simulink model "RocketSimForArchitecture"  (R2024b)
settings: Solver=VariableStepAuto  StartTime=0.0  StopTime=10.0  RelTol=1e-3  AbsTol=1e-3
model workspace (MAT data in the model file):
  m = 1
values from neighbouring files (symbols this model uses):
  X =     [ga_pid_best_result.mat]    (also in pid_vals.mat)
  Y =     [ga_pid_best_result.mat]    (also in pid_vals.mat)
  Z =     [ga_pid_best_result.mat]    (also in pid_vals.mat)
libraries: fl_lib x25, nesl_utility x22, sm_lib x12, ee_lib x9, slpidlib x4, matrix_library x2, aerolibutil x2, sdl_lib x1, shared6dof x1, robotcorelib x1, aerolibnav x1
(part 2 of 2)

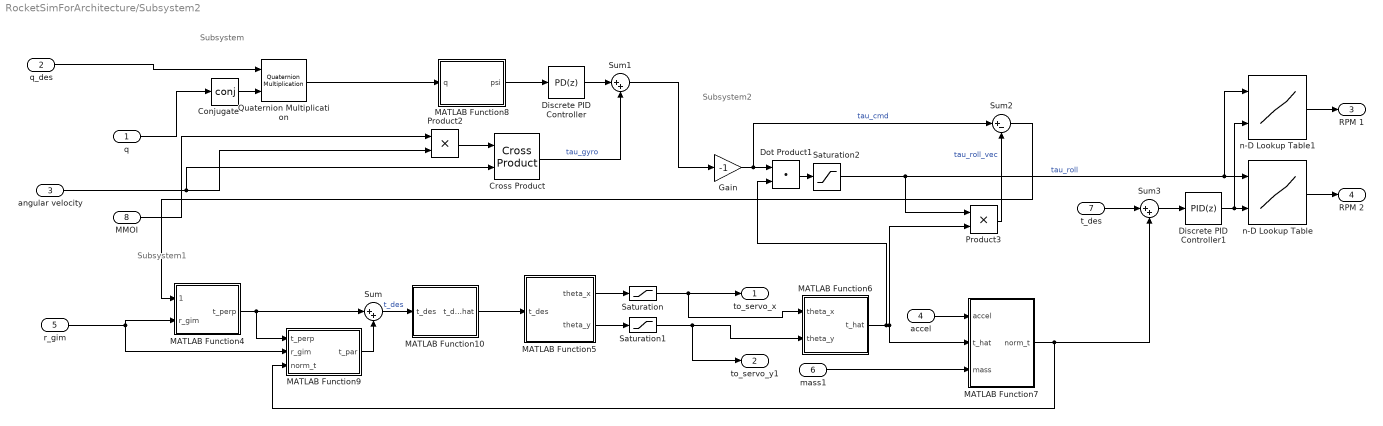
== system RocketSimForArchitecture/Subsystem2 ==
  note: Subsystem1
  note: Subsystem
  note: Subsystem2
  q : Inport  PortDimensions=4
  q_des : Inport  Port=2  PortDimensions=4
  angular velocity : Inport  Port=3  PortDimensions=3
  accel : Inport  Port=4  PortDimensions=3
  r_gim : Inport  Port=5  PortDimensions=3
  mass1 : Inport  Port=6  PortDimensions=1
  t_des : Inport  Port=7  PortDimensions=3
  MMOI : Inport  Port=8
  Conjugate : Math  Operator=conj  SignedPower=on  RndMeth=Zero
  Cross Product : matrix_library/Cross Product
  Discrete PID Controller : slpidlib/PID Controller  Controller=PD  Form=Parallel  TimeDomain=Discrete-time  UseExternalTs=off  SampleTime=0.001  IntegratorMethod=Forward Euler  FilterMethod=Forward Euler  ControllerParametersSource=internal  P=1  I=1  UseKiTs=off  D=1  UseExternalDerivativeSource=off  N=1  UseFilter=on  TunerSelectOption=Transfer Function Based (PID Tuner App)  InitialConditionSource=internal  InitialConditionForIntegrator=0  InitialConditionForFilter=1  DifferentiatorICPrevScaledInput=0  ExternalReset=none  TrackingMode=off  Kt=1  LimitOutput=on  SatLimitsSource=internal  UpperSaturationLimit=10  LowerSaturationLimit=-10  LinearizeAsGain=off  AntiWindupMode=none  Kb=1  LimitIntegrator=off  UpperIntegratorSaturationLimit=inf  LowerIntegratorSaturationLimit=-inf  POutMin=[]  POutMax=[]  IOutMin=[]  IOutMax=[]  DOutMin=[]  DOutMax=[]  NOutMin=[]  NOutMax=[]  SumOutMin=[]  SumOutMax=[]  SaturationOutMin=[]  SaturationOutMax=[]  PParamMin=[]  PParamMax=[]  IParamMin=[]  IParamMax=[]  DParamMin=[]  DParamMax=[]  NParamMin=[]  NParamMax=[]  KbParamMin=[]  KbParamMax=[]  KtParamMin=[]  KtParamMax=[]  KbOutMin=[]  KbOutMax=[]  KtOutMin=[]  KtOutMax=[]  IntegratorOutMin=[]  IntegratorOutMax=[]  FilterOutMin=[]  FilterOutMax=[]  SumI1OutMin=[]  SumI1OutMax=[]  SumI2OutMin=[]  SumI2OutMax=[]  SumI3OutMin=[]  SumI3OutMax=[]  SumI4OutMin=[]  SumI4OutMax=[]  SumDOutMin=[]  SumDOutMax=[]  DifferentiatorOutMin=[]  DifferentiatorOutMax=[]  FilterDiffOutCoefMin=[]  FilterDiffOutCoefMax=[]  ReciprocalOutMin=[]  ReciprocalOutMax=[]  SumDenOutMin=[]  SumDenOutMax=[]  SumNumOutMin=[]  SumNumOutMax=[]  DivideOutMin=[]  DivideOutMax=[]  UdiffTsProdOutMin=[]  UdiffTsProdOutMax=[]  NTsProdOutMin=[]  NTsProdOutMax=[]  UintegralTsProdOutMin=[]  UintegralTsProdOutMax=[]  UngainTsProdOutMin=[]  UngainTsProdOutMax=[]  ClampingZeroOutDataTypeStr=Inherit: Inherit via back propagation  ClampingZeroOutMin=[]  ClampingZeroOutMax=[]  FilterDenConstantOutDataTypeStr=Inherit: Inherit via back propagation  FilterDenConstantOutMin=[]  FilterDenConstantOutMax=[]  PCopyOutDataTypeStr=Inherit: Inherit via back propagation  PCopyOutMin=[]  PCopyOutMax=[]  NCopyOutDataTypeStr=Inherit: Inherit via back propagation  NCopyOutMin=[]  NCopyOutMax=[]  IntegratorContinuousStateAttributes=''  IntegratorStateMustResolveToSignalObject=off  IntegratorRTWStateStorageClass=Auto  FilterContinuousStateAttributes=''  FilterStateMustResolveToSignalObject=off  FilterRTWStateStorageClass=Auto  ParallelPVariant=InternalParameters  IdealPVariant=Disabled  IVariant=Disabled  DVariant=InternalParameters  IntegratorVariant=Disabled  SatVariant=Enabled  AWVariant=Disabled  PCopyVariant=Disabled  TRVariant=Disabled  FdbkBlocksVariant=Forward  IdealPFdbkVariant=Disabled  SatFdbkVariant=Disabled  DerivativeFilterVariant=ForwardEulerFilter  NVariant=InternalParameters  NCopyVariant=Disabled  FilterICVariant=InternalICsFilter  IntegratorICVariant=Disabled  ExternalResetVariant=Disabled  TRSumVariant=Passthrough  SumFdbkVariant=Disabled  SumVariant=Sum_PD  TsampFilterVariant=InternalTs  TsampNgainVariant=Passthrough  TsampIntegralVariant=Disabled_SignalSpec  ExternalSaturationOutDataTypeStr=Inherit: Same as second input  DerivativeSourceVariant=ErrorSignal  PreIntVariant=InternalPreInt
  Discrete PID Controller1 : slpidlib/PID Controller  Controller=PID  Form=Parallel  TimeDomain=Discrete-time  UseExternalTs=off  SampleTime=0.001  IntegratorMethod=Forward Euler  FilterMethod=Forward Euler  ControllerParametersSource=internal  P=0  I=1  UseKiTs=off  D=1  UseExternalDerivativeSource=off  N=100  UseFilter=on  TunerSelectOption=Transfer Function Based (PID Tuner App)  InitialConditionSource=internal  InitialConditionForIntegrator=0  InitialConditionForFilter=0  DifferentiatorICPrevScaledInput=0  ExternalReset=none  TrackingMode=off  Kt=1  LimitOutput=off  SatLimitsSource=internal  UpperSaturationLimit=inf  LowerSaturationLimit=-inf  LinearizeAsGain=off  AntiWindupMode=none  Kb=1  LimitIntegrator=off  UpperIntegratorSaturationLimit=inf  LowerIntegratorSaturationLimit=-inf  POutMin=[]  POutMax=[]  IOutMin=[]  IOutMax=[]  DOutMin=[]  DOutMax=[]  NOutMin=[]  NOutMax=[]  SumOutMin=[]  SumOutMax=[]  SaturationOutMin=[]  SaturationOutMax=[]  PParamMin=[]  PParamMax=[]  IParamMin=[]  IParamMax=[]  DParamMin=[]  DParamMax=[]  NParamMin=[]  NParamMax=[]  KbParamMin=[]  KbParamMax=[]  KtParamMin=[]  KtParamMax=[]  KbOutMin=[]  KbOutMax=[]  KtOutMin=[]  KtOutMax=[]  IntegratorOutMin=[]  IntegratorOutMax=[]  FilterOutMin=[]  FilterOutMax=[]  SumI1OutMin=[]  SumI1OutMax=[]  SumI2OutMin=[]  SumI2OutMax=[]  SumI3OutMin=[]  SumI3OutMax=[]  SumI4OutMin=[]  SumI4OutMax=[]  SumDOutMin=[]  SumDOutMax=[]  DifferentiatorOutMin=[]  DifferentiatorOutMax=[]  FilterDiffOutCoefMin=[]  FilterDiffOutCoefMax=[]  ReciprocalOutMin=[]  ReciprocalOutMax=[]  SumDenOutMin=[]  SumDenOutMax=[]  SumNumOutMin=[]  SumNumOutMax=[]  DivideOutMin=[]  DivideOutMax=[]  UdiffTsProdOutMin=[]  UdiffTsProdOutMax=[]  NTsProdOutMin=[]  NTsProdOutMax=[]  UintegralTsProdOutMin=[]  UintegralTsProdOutMax=[]  UngainTsProdOutMin=[]  UngainTsProdOutMax=[]  ClampingZeroOutDataTypeStr=Inherit: Inherit via back propagation  ClampingZeroOutMin=[]  ClampingZeroOutMax=[]  FilterDenConstantOutDataTypeStr=Inherit: Inherit via back propagation  FilterDenConstantOutMin=[]  FilterDenConstantOutMax=[]  PCopyOutDataTypeStr=Inherit: Inherit via back propagation  PCopyOutMin=[]  PCopyOutMax=[]  NCopyOutDataTypeStr=Inherit: Inherit via back propagation  NCopyOutMin=[]  NCopyOutMax=[]  IntegratorContinuousStateAttributes=''  IntegratorStateMustResolveToSignalObject=off  IntegratorRTWStateStorageClass=Auto  FilterContinuousStateAttributes=''  FilterStateMustResolveToSignalObject=off  FilterRTWStateStorageClass=Auto  ParallelPVariant=InternalParameters  IdealPVariant=Disabled  IVariant=InternalParameters  DVariant=InternalParameters  IntegratorVariant=Discrete  SatVariant=Disabled  AWVariant=Passthrough  PCopyVariant=Disabled  TRVariant=Disabled  FdbkBlocksVariant=Forward  IdealPFdbkVariant=Disabled  SatFdbkVariant=Disabled  DerivativeFilterVariant=ForwardEulerFilter  NVariant=InternalParameters  NCopyVariant=Disabled  FilterICVariant=InternalICsFilter  IntegratorICVariant=InternalICs  ExternalResetVariant=Disabled  TRSumVariant=Passthrough  SumFdbkVariant=Disabled  SumVariant=Sum_PID  TsampFilterVariant=InternalTs  TsampNgainVariant=Passthrough  TsampIntegralVariant=Disabled_SignalSpec  ExternalSaturationOutDataTypeStr=Inherit: Same as second input  DerivativeSourceVariant=ErrorSignal  PreIntVariant=InternalPreInt
  Dot Product1 : DotProduct  OutDataTypeStr=Inherit: Inherit via internal rule
  Gain : Gain  Gain=-1
  MATLAB Function10 : MATLAB Function  TreatAsAtomicUnit=on
  MATLAB Function4 : MATLAB Function  TreatAsAtomicUnit=on
  MATLAB Function5 : MATLAB Function  TreatAsAtomicUnit=on
  MATLAB Function6 : MATLAB Function  TreatAsAtomicUnit=on
  MATLAB Function7 : MATLAB Function  TreatAsAtomicUnit=on
  MATLAB Function8 : MATLAB Function  TreatAsAtomicUnit=on
  MATLAB Function9 : MATLAB Function  TreatAsAtomicUnit=on
  Product2 : Product
  Product3 : Product
  Quaternion Multiplication : aerolibutil/Quaternion Multiplication
  Saturation : Saturate
  Saturation1 : Saturate
  Saturation2 : Saturate
  Sum : Sum  Inputs=|++
  Sum1 : Sum  Inputs=|++
  Sum2 : Sum  Inputs=|+-
  Sum3 : Sum  Inputs=|++
  n-D Lookup Table : Lookup_n-D  LookupTableObject=''  BreakpointsForDimension1=[1:2]  BreakpointsForDimension2=[1:2]  BreakpointsForDimension3=[5, 7]  BreakpointsForDimension1FirstPoint=10  BreakpointsForDimension2FirstPoint=10  BreakpointsForDimension1Spacing=12  BreakpointsForDimension2Spacing=12  IndexSearchMethod=Evenly spaced points  Table=[4 5;16 19]  InterpMethod=Flat  DiagnosticForOutOfRangeInput=Error  InternalRulePriority=Speed  RndMeth=Simplest
      settings: InputPortMap=u0,u1
  n-D Lookup Table1 : Lookup_n-D  LookupTableObject=''  BreakpointsForDimension1=[1:2]  BreakpointsForDimension2=[1:2]  BreakpointsForDimension3=[5, 7]  BreakpointsForDimension1FirstPoint=10  BreakpointsForDimension2FirstPoint=10  BreakpointsForDimension1Spacing=12  BreakpointsForDimension2Spacing=12  IndexSearchMethod=Evenly spaced points  Table=[4 5;16 19]  InterpMethod=Flat  DiagnosticForOutOfRangeInput=Error  InternalRulePriority=Speed  RndMeth=Simplest
      settings: InputPortMap=u0,u1
  to_servo_x : Outport  PortDimensions=1
  to_servo_y1 : Outport  Port=2  PortDimensions=1
  RPM 1 : Outport  Port=3
  RPM 2 : Outport  Port=4
  wires:
  Discrete PID Controller1/1 -> n-D Lookup Table1/2, n-D Lookup Table/2
  Conjugate/1 -> Quaternion Multiplication/2
  MATLAB Function5/1(theta_x) -> Saturation/1
  Quaternion Multiplication/1 -> MATLAB Function8/1(q)
  Gain/1 -> Sum2/1, Dot Product1/1  "tau_cmd"
  n-D Lookup Table/1 -> RPM 2/1
  Saturation1/1 -> to_servo_y1/1, MATLAB Function6/2(theta_y)
  Sum/1 -> MATLAB Function10/1(t_des)  "t_des"
  Saturation/1 -> to_servo_x/1, MATLAB Function6/1(theta_x)
  Dot Product1/1 -> Saturation2/1
  accel/1 -> MATLAB Function7/1(accel)
  Cross Product/1 -> Sum1/2  "tau_gyro"
  MATLAB Function6/1(t_hat) -> Product3/2, MATLAB Function7/2(t_hat), Dot Product1/2
  MMOI/1 -> Product2/1
  Sum2/1 -> MATLAB Function4/1(tau_gim)
  MATLAB Function4/1(t_perp) -> MATLAB Function9/1(t_perp), Sum/1
  mass1/1 -> MATLAB Function7/3(mass)
  MATLAB Function10/1(t_des_hat) -> MATLAB Function5/1(t_des)
  MATLAB Function5/2(theta_y) -> Saturation1/1
  r_gim/1 -> MATLAB Function9/2(r_gim), MATLAB Function4/2(r_gim)
  q_des/1 -> Quaternion Multiplication/1
  Saturation2/1 -> n-D Lookup Table1/1, n-D Lookup Table/1, Product3/1  "tau_roll"
  angular velocity/1 -> Product2/2, Cross Product/2
  MATLAB Function8/1(psi) -> Discrete PID Controller/1
  MATLAB Function7/1(norm_t) -> MATLAB Function9/3(norm_t), Sum3/2
  Product3/1 -> Sum2/2  "tau_roll_vec"
  Sum1/1 -> Gain/1
  Sum3/1 -> Discrete PID Controller1/1
  q/1 -> Conjugate/1
  Discrete PID Controller/1 -> Sum1/1
  MATLAB Function9/1(t_par) -> Sum/2
  Product2/1 -> Cross Product/1
  t_des/1 -> Sum3/1
  n-D Lookup Table1/1 -> RPM 1/1

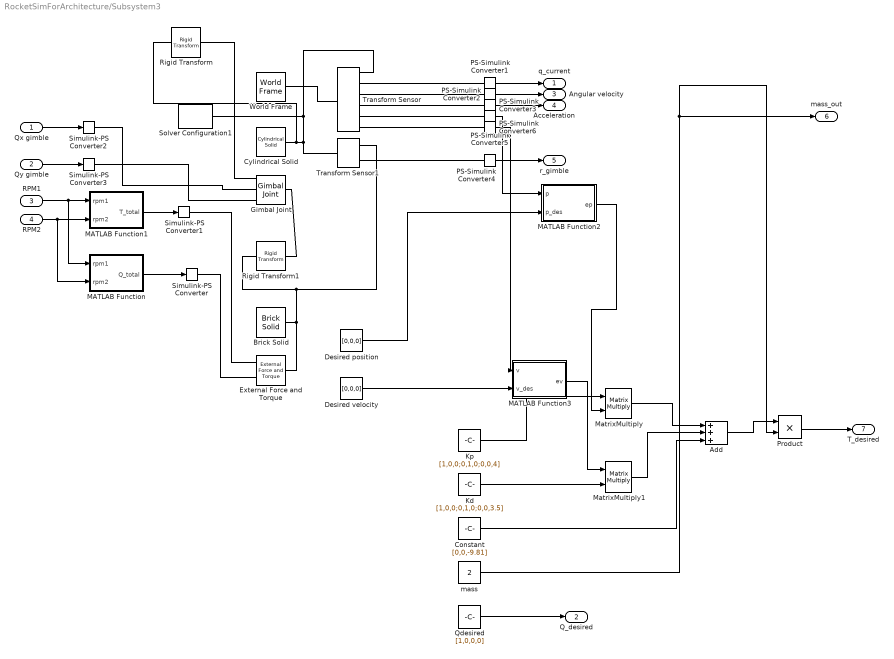
== system RocketSimForArchitecture/Subsystem3 ==
  Qx gimble : Inport
  Qy gimble : Inport  Port=2
  RPM1 : Inport  Port=3
  RPM2 : Inport  Port=4
  Add : Sum  Inputs=+++
  Brick Solid : sm_lib/Body Elements/Brick Solid  BrickDimensions=[0.1 0.1 0.2]  BrickDimensionsUnits=m  ExportEntireGeometry=off  InertiaType=CalculateFromGeometry  BasedOnType=Mass  Density=1000  DensityUnits=kg/m^3  Mass=0.5  MassUnits=kg  CenterOfMass=[0 0 0]  CenterOfMassUnits=m  MomentsOfInertia=[1 1 1]  MomentsOfInertiaUnits=kg*m^2  ProductsOfInertia=[0 0 0]  ProductsOfInertiaUnits=kg*m^2  GraphicType=FromGeometry  MarkerShape=Sphere  MarkerSize=10  GraphicVisPropType=SimpleVisualProperties  GraphicDiffuseColor=[1 0 0]  GraphicOpacity=1  GraphicSpecularColor=[0.5 0.5 0.5 1.0]  GraphicAmbientColor=[0.15 0.15 0.15 1.0]  GraphicEmissiveColor=[0.0 0.0 0.0 1.0]  GraphicShininess=75  DoExposeReferenceFrame=on  SerializedFrames=<Frames/>
  Constant : Constant  Value=[0,0,-9.81]
  Cylindrical Solid : sm_lib/Body Elements/Cylindrical Solid  CylinderRadius=0.08  CylinderRadiusUnits=m  CylinderLength=0.4  CylinderLengthUnits=m  ExportEntireGeometry=off  InertiaType=CalculateFromGeometry  BasedOnType=Mass  Density=1.5  DensityUnits=kg/m^3  Mass=1.5  MassUnits=kg  CenterOfMass=[0 0 0]  CenterOfMassUnits=m  MomentsOfInertia=[1 1 1]  MomentsOfInertiaUnits=kg*m^2  ProductsOfInertia=[0 0 0]  ProductsOfInertiaUnits=kg*m^2  GraphicType=FromGeometry  MarkerShape=Sphere  MarkerSize=10  GraphicVisPropType=SimpleVisualProperties  GraphicDiffuseColor=[0 0.4471 0.7412]  GraphicOpacity=1  GraphicSpecularColor=[0.5 0.5 0.5 1.0]  GraphicAmbientColor=[0.15 0.15 0.15 1.0]  GraphicEmissiveColor=[0.0 0.0 0.0 1.0]  GraphicShininess=75  DoExposeReferenceFrame=on  SerializedFrames=<Frames/>
  Desired position : Constant  Value=[0,0,0]
  Desired velocity : Constant  Value=[0,0,0]
  External Force and Torque : sm_lib/Forces and Torques/External Force and Torque  EnableForceX=off  EnableForceY=off  EnableForceZ=on  EnableForce=off  ForceResolutionFrame=AttachedFrame  EnableTorqueX=off  EnableTorqueY=off  EnableTorqueZ=on  EnableTorque=off  TorqueResolutionFrame=AttachedFrame
  Gimbal Joint : sm_lib/Joints/Gimbal Joint  JointMode=Normal  CompositeWrenchDir=FollowerOnBase  CompositeWrenchFrame=BaseFrame  SenseConstraintForce=off  SenseConstraintTorque=off  SenseTotalForce=off  SenseTotalTorque=off  RxPositionTargetSpecify=off  RxPositionTargetPriority=High  RxPositionTargetValue=0  RxPositionTargetValueUnits=deg  RxVelocityTargetSpecify=off  RxVelocityTargetPriority=High  RxVelocityTargetValue=0  RxVelocityTargetValueUnits=deg/s  RxEquilibriumPosition=0  RxEquilibriumPositionUnits=deg  RxSpringStiffness=0  RxSpringStiffnessUnits=N*m/deg  RxDampingCoefficient=0  RxDampingCoefficientUnits=N*m/(deg/s)  RxLowerLimitSpecify=off  RxLowerLimitBound=-90  RxLowerLimitBoundUnits=deg  RxLowerLimitStiffness=1e4  RxLowerLimitStiffnessUnits=N*m/deg  RxLowerLimitDamping=10  RxLowerLimitDampingUnits=N*m/(deg/s)  RxLowerLimitTransitionRegionWidth=0.1  RxLowerLimitTransitionRegionWidthUnits=deg  RxUpperLimitSpecify=off  RxUpperLimitBound=90  RxUpperLimitBoundUnits=deg  RxUpperLimitStiffness=1e4  RxUpperLimitStiffnessUnits=N*m/deg  RxUpperLimitDamping=10  RxUpperLimitDampingUnits=N*m/(deg/s)  RxUpperLimitTransitionRegionWidth=0.1  RxUpperLimitTransitionRegionWidthUnits=deg  RxTorqueActuationMode=ComputedTorque  RxMotionActuationMode=InputMotion  RxSensePosition=off  RxSenseVelocity=off  RxSenseAcceleration=off  RxSenseTorqueForce=off  RxSenseLowerLimitTorqueForce=off  RxSenseUpperLimitTorqueForce=off  RyPositionTargetSpecify=off  RyPositionTargetPriority=High  RyPositionTargetValue=0  RyPositionTargetValueUnits=deg  RyVelocityTargetSpecify=off  RyVelocityTargetPriority=High  RyVelocityTargetValue=0  RyVelocityTargetValueUnits=deg/s  RyEquilibriumPosition=0  RyEquilibriumPositionUnits=deg  RySpringStiffness=0  RySpringStiffnessUnits=N*m/deg  RyDampingCoefficient=0  RyDampingCoefficientUnits=N*m/(deg/s)  RyLowerLimitSpecify=off  RyLowerLimitBound=-90  RyLowerLimitBoundUnits=deg  RyLowerLimitStiffness=1e4  RyLowerLimitStiffnessUnits=N*m/deg  RyLowerLimitDamping=10  RyLowerLimitDampingUnits=N*m/(deg/s)  RyLowerLimitTransitionRegionWidth=0.1  RyLowerLimitTransitionRegionWidthUnits=deg  RyUpperLimitSpecify=off  RyUpperLimitBound=90  RyUpperLimitBoundUnits=deg  RyUpperLimitStiffness=1e4  RyUpperLimitStiffnessUnits=N*m/deg  RyUpperLimitDamping=10  RyUpperLimitDampingUnits=N*m/(deg/s)  RyUpperLimitTransitionRegionWidth=0.1  RyUpperLimitTransitionRegionWidthUnits=deg  RyTorqueActuationMode=NoTorque  RyMotionActuationMode=InputMotion  RySensePosition=off  RySenseVelocity=off  RySenseAcceleration=off  RySenseTorqueForce=off  RySenseLowerLimitTorqueForce=off  RySenseUpperLimitTorqueForce=off  RzPositionTargetSpecify=off  RzPositionTargetPriority=High  RzPositionTargetValue=0  RzPositionTargetValueUnits=deg  RzVelocityTargetSpecify=off  RzVelocityTargetPriority=High  RzVelocityTargetValue=0  RzVelocityTargetValueUnits=deg/s  RzEquilibriumPosition=0  RzEquilibriumPositionUnits=deg  RzSpringStiffness=0  RzSpringStiffnessUnits=N*m/deg  RzDampingCoefficient=0  RzDampingCoefficientUnits=N*m/(deg/s)  RzLowerLimitSpecify=off  RzLowerLimitBound=-90  RzLowerLimitBoundUnits=deg  RzLowerLimitStiffness=1e4  RzLowerLimitStiffnessUnits=N*m/deg  RzLowerLimitDamping=10  RzLowerLimitDampingUnits=N*m/(deg/s)  RzLowerLimitTransitionRegionWidth=0.1  RzLowerLimitTransitionRegionWidthUnits=deg  RzUpperLimitSpecify=off  RzUpperLimitBound=90  RzUpperLimitBoundUnits=deg  RzUpperLimitStiffness=1e4  RzUpperLimitStiffnessUnits=N*m/deg  RzUpperLimitDamping=10  RzUpperLimitDampingUnits=N*m/(deg/s)  RzUpperLimitTransitionRegionWidth=0.1  RzUpperLimitTransitionRegionWidthUnits=deg  RzTorqueActuationMode=NoTorque  RzMotionActuationMode=ComputedMotion  RzSensePosition=off  RzSenseVelocity=off  RzSenseAcceleration=off  RzSenseTorqueForce=off  RzSenseLowerLimitTorqueForce=off  RzSenseUpperLimitTorqueForce=off
  Kd : Constant  Value=[1,0,0;0,1,0;0,0,3.5]
  Kp : Constant  Value=[1,0,0;0,1,0;0,0,4]
  MATLAB Function : MATLAB Function  TreatAsAtomicUnit=on
  MATLAB Function1 : MATLAB Function  TreatAsAtomicUnit=on
  MATLAB Function2 : MATLAB Function  TreatAsAtomicUnit=on
  MATLAB Function3 : MATLAB Function  TreatAsAtomicUnit=on
  MatrixMultiply : Product  Multiplication=Matrix(*)
  MatrixMultiply1 : Product  Multiplication=Matrix(*)
  PS-Simulink Converter{1..6} (6 alike) : nesl_utility/PS-Simulink Converter  PhysicalDomain=network_engine_domain  SubClassName=ps_output  LeftPortType=input  RightPortType=output  PseudoPeriodic=off  Frequencies=[]  VectorFormat=inherit  Unit=inherit  AffineConversion=off
  Product : Product
  Qdesired : Constant  Value=[1,0,0,0]
  Rigid Transform : sm_lib/Frames and Transforms/Rigid Transform  RotationMethod=None  FollAlignAxisA=+X  BaseAlignAxisA=+Y  FollAlignAxisB=+Y  BaseAlignAxisB=+Z  RotationStandardAxis=+Z  RotationAngle=0  RotationAngleUnits=deg  RotationArbitraryAxis=[0 0 1]  RotationSequenceAxes=FollowerAxes  RotationSequence=XYX  RotationSequenceAngles=[0 0 0]  RotationSequenceAnglesUnits=deg  RotationMatrix=[1 0 0;0 1 0;0 0 1]  Quaternion=[1 0 0 0]  TranslationMethod=Cartesian  TranslationCartesianOffset=[0 0 -0.2]  TranslationCartesianOffsetUnits=m  TranslationStandardAxis=+Z  TranslationStandardOffset=0  TranslationStandardOffsetUnits=m  TranslationROffset=0  TranslationROffsetUnits=m  TranslationThetaOffset=0  TranslationThetaOffsetUnits=deg  TranslationZOffset=0  TranslationZOffsetUnits=m
  Rigid Transform1 : sm_lib/Frames and Transforms/Rigid Transform  RotationMethod=None  FollAlignAxisA=+X  BaseAlignAxisA=+Y  FollAlignAxisB=+Y  BaseAlignAxisB=+Z  RotationStandardAxis=+Z  RotationAngle=0  RotationAngleUnits=deg  RotationArbitraryAxis=[0 0 1]  RotationSequenceAxes=FollowerAxes  RotationSequence=XYX  RotationSequenceAngles=[0 0 0]  RotationSequenceAnglesUnits=deg  RotationMatrix=[1 0 0;0 1 0;0 0 1]  Quaternion=[1 0 0 0]  TranslationMethod=Cartesian  TranslationCartesianOffset=[0 0 0.1]  TranslationCartesianOffsetUnits=m  TranslationStandardAxis=+Z  TranslationStandardOffset=0  TranslationStandardOffsetUnits=m  TranslationROffset=0  TranslationROffsetUnits=m  TranslationThetaOffset=0  TranslationThetaOffsetUnits=deg  TranslationZOffset=0  TranslationZOffsetUnits=m
  Simulink-PS Converter{,1..3} (4 alike) : nesl_utility/Simulink-PS Converter  PhysicalDomain=network_engine_domain  SubClassName=ps_input  LeftPortType=input  RightPortType=output  PseudoPeriodic=off  Frequencies=[]  NoiseDistribution=none  NoiseParameters=[]  Unit=1  AffineConversion=off  FilteringAndDerivatives=provide  SimscapeFilterOrder=1  InputFilterTimeConstant=0.001  UdotUserProvided=0
  Solver Configuration1 : nesl_utility/Solver Configuration  PhysicalDomain=network_engine_domain  SubClassName=solver  LeftPortType=input  RightPortType=generic  Tones=[]  Harmonics=[]  SimulateNoise=off  Profile=off  UseLocalSampling=off  EnableSwitchedLinearOptims=on  FrequencyDomain=off  UseCCode=off  RelTol=0.001  AbsTol=0.001  MinStep=1e-09  ToWorkspace=off  RevertToSquareIcSolve=off  NumHomotopyIterations=100  PhasorMode=off  PhasorModeNumHarmonics=1  ConsistencySolver=NEWTON_XTOL_AFTER_FTOL  IndexReductionMethod=DerivativeReplacement  DoDC=off  ResidualTolerance=1e-09  ConsistencyTolSource=GLOBAL  ConsistencyAbsTol=0.001  ConsistencyRelTol=0.001  ConsistencyTolFactor=0.001  UseLocalSolver=off  LocalSolverChoice=NE_BACKWARD_EULER_ADVANCER  ResolveIndetEquations=on  FunctionEvalNumThread=1  LocalSolverSampleTime=0.001  DoFixedCost=off  MaxNonlinIter=3  MaxModeIter=2  ComputeImpulses=off  ImpulseIterations=2  LinearAlgebra=auto  LinearAlgebraNumThread=0  EquationFormulation=NE_TIME_EF  DelaysMemoryBudget=1024  AutomaticFiltering=on  FilteringTimeConstant=0.001  PartitionStorageMethod=AS_NEEDED  PartitionMemoryBudget=1024  PartitionMethod=ROBUST  MultibodyUseLocalSolver=on  MultibodyLocalSolverChoice=ODE1  MultibodyLocalSolverSampleTime=0.001
  Transform Sensor : sm_lib/Frames and Transforms/Transform Sensor  MeasurementFrame=World  RotationSequence=XYX  SenseAngle=off  SenseAxis=off  SenseQ=on  SenseR=off  SenseRotationSequence=off  SenseOmegaX=off  SenseOmegaY=off  SenseOmegaZ=off  SenseOmega=on  SenseQDot=off  SenseRDot=off  SenseRotationSequenceDot=off  SenseAlphaX=off  SenseAlphaY=off  SenseAlphaZ=off  SenseAlpha=off  SenseQDDot=off  SenseRDDot=off  SenseX=off  SenseY=off  SenseZ=off  SenseXYZ=on  SenseRad=off  SenseAzim=off  SenseDist=off  SenseInc=off  SenseXDot=off  SenseYDot=off  SenseZDot=off  SenseXYZDot=on  SenseRadDot=off  SenseAzimDot=off  SenseDistDot=off  SenseIncDot=off  SenseXDDot=off  SenseYDDot=off  SenseZDDot=off  SenseXYZDDot=on  SenseRadDDot=off  SenseAzimDDot=off  SenseDistDDot=off  SenseIncDDot=off
  Transform Sensor1 : sm_lib/Frames and Transforms/Transform Sensor  MeasurementFrame=World  RotationSequence=XYX  SenseAngle=off  SenseAxis=off  SenseQ=off  SenseR=off  SenseRotationSequence=off  SenseOmegaX=off  SenseOmegaY=off  SenseOmegaZ=off  SenseOmega=off  SenseQDot=off  SenseRDot=off  SenseRotationSequenceDot=off  SenseAlphaX=off  SenseAlphaY=off  SenseAlphaZ=off  SenseAlpha=off  SenseQDDot=off  SenseRDDot=off  SenseX=off  SenseY=off  SenseZ=off  SenseXYZ=on  SenseRad=off  SenseAzim=off  SenseDist=off  SenseInc=off  SenseXDot=off  SenseYDot=off  SenseZDot=off  SenseXYZDot=off  SenseRadDot=off  SenseAzimDot=off  SenseDistDot=off  SenseIncDot=off  SenseXDDot=off  SenseYDDot=off  SenseZDDot=off  SenseXYZDDot=off  SenseRadDDot=off  SenseAzimDDot=off  SenseDistDDot=off  SenseIncDDot=off
  World Frame : sm_lib/Frames and Transforms/World Frame
  mass : Constant  Value=2
  q_current : Outport
  Q_desired : Outport  Port=2
  Angular velocity : Outport  Port=3
  Acceleration : Outport  Port=4
  r_gimble : Outport  Port=5
  mass_out : Outport  Port=6
  T_desired : Outport  Port=7
  wires:
  Qx gimble/1 -> Simulink-PS Converter2/1
  MATLAB Function2/1(ep) -> MatrixMultiply/2
  PS-Simulink Converter3/1 -> Acceleration/1
  MATLAB Function/1(Q_total) -> Simulink-PS Converter/1
  Desired velocity/1 -> MATLAB Function3/2(v_des)
  Kd/1 -> MatrixMultiply1/2
  PS-Simulink Converter4/1 -> r_gimble/1
  MatrixMultiply/1 -> Add/1
  MATLAB Function3/1(ev) -> MatrixMultiply1/1
  Qdesired/1 -> Q_desired/1
  PS-Simulink Converter1/1 -> q_current/1
  PS-Simulink Converter2/1 -> Angular velocity/1
  PS-Simulink Converter6/1 -> MATLAB Function3/1(v)
  Add/1 -> Product/1
  MATLAB Function1/1(T_total) -> Simulink-PS Converter1/1
  Qy gimble/1 -> Simulink-PS Converter3/1
  Kp/1 -> MatrixMultiply/1
  mass/1 -> Product/2, mass_out/1
  Constant/1 -> Add/3
  RPM2/1 -> MATLAB Function/2(rpm2), MATLAB Function1/2(rpm2)
  Desired position/1 -> MATLAB Function2/2(p_des)
  MatrixMultiply1/1 -> Add/2
  PS-Simulink Converter5/1 -> MATLAB Function2/1(p)
  Product/1 -> T_desired/1
  RPM1/1 -> MATLAB Function/1(rpm1), MATLAB Function1/1(rpm1)
  connections:
  PS-Simulink Converter3/LConn1 -- Transform Sensor/RConn4
  Simulink-PS Converter3/RConn1 -- Gimbal Joint/LConn3
  Rigid Transform/RConn1 -- Gimbal Joint/LConn1
  Brick Solid/RConn1 -- External Force and Torque/RConn1 -- Transform Sensor1/RConn1 -- Rigid Transform1/LConn1
  PS-Simulink Converter5/LConn1 -- Transform Sensor/RConn5
  Simulink-PS Converter2/RConn1 -- Gimbal Joint/LConn2
  World Frame/RConn1 -- Transform Sensor/LConn1
  Transform Sensor1/RConn2 -- PS-Simulink Converter4/LConn1
  Simulink-PS Converter1/RConn1 -- External Force and Torque/LConn1
  Transform Sensor1/LConn1 -- Rigid Transform/LConn1 -- Cylindrical Solid/RConn1 -- Solver Configuration1/RConn1 -- Transform Sensor/RConn1
  Rigid Transform1/RConn1 -- Gimbal Joint/RConn1
  PS-Simulink Converter6/LConn1 -- Transform Sensor/RConn6
  PS-Simulink Converter2/LConn1 -- Transform Sensor/RConn3
  Transform Sensor/RConn2 -- PS-Simulink Converter1/LConn1
  Simulink-PS Converter/RConn1 -- External Force and Torque/LConn2

== matlab function RocketSimForArchitecture/Error Control /MATLAB Function5 ==
  data: accel input; norm_t output; t_hat input; mass input
function norm_t = fcn(accel, t_hat, mass)

norm_t = mass*(dot(accel, t_hat));

== matlab function RocketSimForArchitecture/Error Control /MATLAB Function6 ==
  data: q input; psi output
function psi  = fcn(q)

q_0 = q(1);
v = [q(2)
    q(3)
    q(4)];
psi_comp = 2*atan2(norm(v), q_0)*v/norm(v);
psi = sign(psi_comp).*psi_comp;

== matlab function RocketSimForArchitecture/Subsystem3/MATLAB Function1 ==
  data: rpm1 input; T_total output; rpm2 input
function T_total = prop_total_thrust(rpm1, rpm2)
% Outputs only total thrust from two stacked propellers

% --- Coefficients ---
kT  = 1.2e-7;    % thrust coefficient
kQ  = 2.0e-9;    % torque coefficient (unused here)
eta = 0.9;       % efficiency for 2nd prop

% --- Thrust calculations ---
T1 = kT * rpm1^2;
T2 = kT * rpm2^2 * eta;

T_total = T1 + T2;
end

== matlab function RocketSimForArchitecture/Subsystem2/MATLAB Function7 ==
  data: accel input; norm_t output; t_hat input; mass input
function norm_t = fcn(accel, t_hat, mass)

norm_t = mass*(dot(accel, t_hat));

== matlab function RocketSimForArchitecture/Subsystem2/MATLAB Function8 ==
  data: q input; psi output
function psi  = fcn(q)

q_0 = q(1);
v = [q(2)
    q(3)
    q(4)];
psi_comp = 2*atan2(norm(v), q_0)*v/norm(v);
psi = sign(psi_comp).*psi_comp;

== matlab function RocketSimForArchitecture/Error Control /MATLAB Function9 ==
  data: t_perp input; t_par output; r_gim input; norm_t input
function t_par = fcn(t_perp, r_gim, norm_t)

t_par = sqrt(norm_t^2 - norm(t_perp)^2)*r_gim/norm(r_gim);

== matlab function RocketSimForArchitecture/Subsystem2/MATLAB Function9 ==
  data: t_perp input; t_par output; r_gim input; norm_t input
function t_par = fcn(t_perp, r_gim, norm_t)

t_par = sqrt(norm_t^2 - norm(t_perp)^2)*r_gim/norm(r_gim);

== matlab function RocketSimForArchitecture/Subsystem3/MATLAB Function ==
  data: rpm1 input; Q_total output; rpm2 input
function Q_total = prop_total_torque(rpm1, rpm2)
% Outputs only total torque from two stacked propellers

% --- Coefficients ---
kT  = 1.2e-7;     % thrust coefficient (unused here)
kQ  = 2.0e-9;     % torque coefficient
eta = 0.9;        % efficiency for 2nd prop

% --- Torque calculations ---
Q1 = -kQ * rpm1^2;           % CW rotation
Q2 =  kQ * rpm2^2 * eta;     % CCW rotation

Q_total = Q1 + Q2;
end

== matlab function RocketSimForArchitecture/Subsystem3/MATLAB Function2 ==
  data: p input; ep output; p_des input
function ep = fcn(p, p_des)

ep = p_des -p;

== matlab function RocketSimForArchitecture/Subsystem3/MATLAB Function3 ==
  data: v input; ev output; v_des input
function ev = fcn(v, v_des)

ev = v_des -v;

== matlab function RocketSimForArchitecture/Subsystem2/MATLAB Function10 ==
  data: t_des input; t_des_hat output
function t_des_hat = fcn(t_des)
t_des_hat = t_des/norm(t_des);

== matlab function RocketSimForArchitecture/Subsystem2/MATLAB Function4 ==
  data: tau_gim input; t_perp output; r_gim input
function t_perp = fcn(tau_gim, r_gim)

t_perp = (cross(tau_gim, r_gim))/(norm(r_gim)^2);

== matlab function RocketSimForArchitecture/Subsystem2/MATLAB Function5 ==
  data: t_des input; theta_x output; theta_y output
function [theta_x, theta_y] = fcn(t_des)

%theta_x = -atan2(t_des(2), t_des(3)); % t_des(2) and (3) are y and z axes
%theta_y = asin(t_des(1)); % t_des(1) is on x axis 
theta_x = 1;
theta_y = 1;

== matlab function RocketSimForArchitecture/Subsystem2/MATLAB Function6 ==
  data: theta_x input; t_hat output; theta_y input
function t_hat  = fcn(theta_x, theta_y)

t_hat = [sin(theta_y)
    -sin(theta_x)*cos(theta_y)
    cos(theta_x)*cos(theta_y)];

== matlab function RocketSimForArchitecture/Error Control /MATLAB Function1 ==
  data: tau_gim input; t_perp output; r_gim input
function t_perp = fcn(tau_gim, r_gim)

t_perp = (cross(tau_gim, r_gim))/(norm(r_gim)^2);

== matlab function RocketSimForArchitecture/Error Control /MATLAB Function10 ==
  data: t_des input; t_des_hat output
function t_des_hat = fcn(t_des)
t_des_hat = t_des/norm(t_des);

== matlab function RocketSimForArchitecture/Error Control /MATLAB Function2 ==
  data: t_des input; theta_x output; theta_y output
function [theta_x, theta_y] = fcn(t_des)

%theta_x = -atan2(t_des(2), t_des(3)); % t_des(2) and (3) are y and z axes
%theta_y = asin(t_des(1)); % t_des(1) is on x axis 
theta_x = 1;
theta_y = 1;

== matlab function RocketSimForArchitecture/Error Control /MATLAB Function4 ==
  data: theta_x input; t_hat output; theta_y input
function t_hat  = fcn(theta_x, theta_y)

t_hat = [sin(theta_y)
    -sin(theta_x)*cos(theta_y)
    cos(theta_x)*cos(theta_y)];
